simulink model "lead_compensator_with_disturbance"  (R2023b)
settings: Solver=VariableStepAuto  StartTime=0.0  StopTime=0.05  RelTol=1e-3
libraries: simulink x2
settings Model: Creator=kijun  LastModifiedBy=kijun

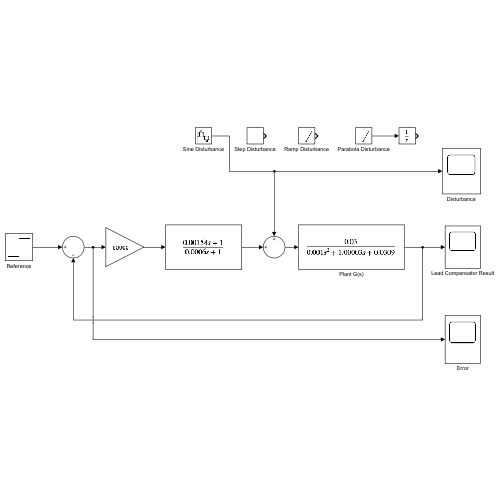
[thumbnail: Simulink's stored preview of the top-level diagram]
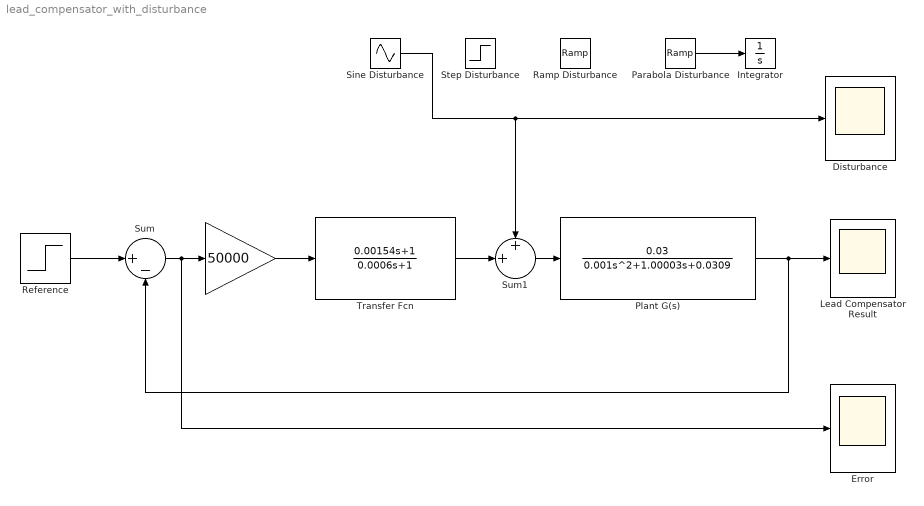
== system lead_compensator_with_disturbance ==
  " " : Gain  Gain=50000
  Disturbance : Scope
  Error : Scope
  Integrator : Integrator
  Lead Compensator Result : Scope
  Parabola Disturbance : simulink/Sources/Ramp  slope=10  start=0  InitialOutput=0
  Plant G(s) : TransferFcn  Numerator=[0.03]  Denominator=[0.001 1.00003 0.0309]
  Ramp Disturbance : simulink/Sources/Ramp  slope=1  start=0  InitialOutput=0
  Reference : Step  Time=0  SampleTime=0
  Sine Disturbance : Sin  Frequency=1000  SampleTime=0.00001
  Step Disturbance : Step  Time=0  SampleTime=0
  Sum : Sum  Inputs=|+-
  Sum1 : Sum  Inputs=++|
  Transfer Fcn : TransferFcn  Numerator=[0.00154 1]  Denominator=[0.0006 1]
  wires:
  Reference/1 -> Sum/1
  Sum/1 -> Error/1, " "/1
  Plant G(s)/1 -> Lead Compensator Result/1, Sum/2
  Transfer Fcn/1 -> Sum1/2
  " "/1 -> Transfer Fcn/1
  Sine Disturbance/1 -> Disturbance/1, Sum1/1
  Parabola Disturbance/1 -> Integrator/1
  Sum1/1 -> Plant G(s)/1
